simulink model "WaypointFollowing_Sim"  (R2021a)
settings: Solver=ode4  StartTime=0.0  StopTime=200  FixedStep=0.001  RelTol=1e-3
InitFcn:
  | Init_control;
values from neighbouring files (symbols this model uses):
  DEG2RAD = 0.0174533    [Init_control.m]
  Kd_PITCH_AngleRate = 0.001    [Init_control.m]
  Kd_ROLL_AngleRate = 0.001    [Init_control.m]
  Kd_YAW_AngleRate = 0.00    (= 0)    [Init_control.m]
  Ki_PITCH_AngleRate = 0.02    [Init_control.m]
  Ki_ROLL_AngleRate = 0.02    [Init_control.m]
  Ki_YAW_AngleRate = 0.01    [Init_control.m]
  Kp_PITCH_ANGLE = 6.5    [Init_control.m]
  Kp_PITCH_AngleRate = 0.1    [Init_control.m]
  Kp_ROLL_ANGLE = 6.5    [Init_control.m]
  Kp_ROLL_AngleRate = 0.1    [Init_control.m]
  Kp_YAW_AngleRate = 0.5    [Init_control.m]
  Kpxp = 1.0    (= 1)    [Init_control.m]
  Kpyp = 1.0    (= 1)    [Init_control.m]
  Kpzp = 4.0    (= 4)    [Init_control.m]
  Kvxd = 0.01    [Init_control.m]
  Kvxi = 0.4    [Init_control.m]
  Kvxp = 2.5    [Init_control.m]
  Kvyd = 0.01    [Init_control.m]
  Kvyi = 0.4    [Init_control.m]
  Kvyp = 2.5    [Init_control.m]
  Kvzd = 0.005    [Init_control.m]
  Kvzi = 0.01    [Init_control.m]
  Kvzp = 0.45    [Init_control.m]
  MAX_CONTROL_ANGLE_PITCH = 35    [Init_control.m]
  MAX_CONTROL_ANGLE_RATE_PITCH = 220    [Init_control.m]
  MAX_CONTROL_ANGLE_RATE_ROLL = 220    [Init_control.m]
  MAX_CONTROL_ANGLE_RATE_Y = 200    [Init_control.m]
  MAX_CONTROL_ANGLE_ROLL = 35    [Init_control.m]
  MAX_CONTROL_VELOCITY_XY = 5    [Init_control.m]
  MAX_CONTROL_VELOCITY_Z = 3    [Init_control.m]
  ModelInit_AngEuler = [0, 0, 0]    [Init_control.m]
  ModelInit_PosE = [0, 0, -100]    [Init_control.m]
  ModelInit_Rads = 0    [Init_control.m]
  ModelInit_RateB = [0, 0, 0]    [Init_control.m]
  ModelInit_VelB = [0, 0, 0]    [Init_control.m]
  Saturation_I_ah = 3.43    [Init_control.m]
  Saturation_I_az = 5    [Init_control.m]
  Saturation_I_RP_Max = 0.3    [Init_control.m]
  Saturation_I_RP_Min = -0.3    [Init_control.m]
  Saturation_I_Y_Max = 0.2    [Init_control.m]
  Saturation_I_Y_Min = -0.2    [Init_control.m]
  THR_HOVER = 0.609    [Init_control.m]
undefined symbols (not defined in the file or in its folder): DiscIntNeverNeededParam, earthRadius, ModelParam_envGravityAcc, ModelParam_motorCr, ModelParam_motorJm, ModelParam_motorT, ModelParam_motorWb, ModelParam_rotorCm, ModelParam_rotorCt, ModelParam_uavCCm, ModelParam_uavCd, ModelParam_uavJ, ModelParam_uavMass, ModelParam_uavR, Receive, Send
libraries: simulink x8, aerolibfltsims x3, sharedutil x2, aerolibanimutils x1
(part 2 of 2)

== matlab function WaypointFollowing_Sim/Quadcopter Dynamics/Rigid Model/Rigid-Body Kinematic Model /Quaternion to rotation matrix ==
  data: q input; Reb output
function Reb = fcn(q)
%Function description;
%  The rotation matrix of the Aircraft-Body Coordinate Frame (ABCF) to the
%  Earth-Fixed Coordinate Frame (EFCF) is obtained from the quaternions
Reb = [q(1)*q(1) + q(2)*q(2) - q(3)*q(3) - q(4)*q(4), 2*(q(2)*q(3) - q(1)*q(4)), 2*(q(2)*q(4) + q(1)*q(3))
           2*(q(2)*q(3) + q(1)*q(4)), q(1)*q(1) - q(2)*q(2) + q(3)*q(3) - q(4)*q(4), 2*(q(3)*q(4) - q(1)*q(2))
           2*(q(2)*q(4) - q(1)*q(3)), 2*(q(3)*q(4) + q(1)*q(2)), q(1)*q(1) - q(2)*q(2) - q(3)*q(3) + q(4)*q(4)];

== matlab function WaypointFollowing_Sim/Quadcopter Dynamics/Rigid Model/Rigid-Body Kinematic Model /Quaternions model ==
  data: pqr input; qdot output; q input
function qdot = fcn(pqr, q)
%Function description:
%  Quaternions model
qdot = 0.5*[0, -pqr(1), -pqr(2), -pqr(3); pqr(1), 0, pqr(3), -pqr(2); pqr(2), -pqr(3), 0, pqr(1); pqr(3), pqr(2), -pqr(1), 0]*q;

== matlab function WaypointFollowing_Sim/Control System/InputConditioning1/f1 ==
  data: in input; y output; hover input
function y = thr_curve(in, hover)
%Function description:
%  throttle curve. When the throttle is in the middle position, the output
%  is hovering throttle value.
%Input:
%  in: normalized throttle, range from 0 to 1
%  hover: hovering throttle value
%Output:
%  y: processed throttle value
if in < 0.5
	y=2 * in * hover;
else
	y=hover + 2 * (in - 0.5) * (1.0 - hover);
end

== matlab function WaypointFollowing_Sim/Control System/MATLAB Function1 ==
  data: reset_i output; ch3 input
function reset_i= fcn(ch3)
%Function description:
%  Reset Integral when throttle < 1250
if ch3<1250
    reset_i=[1 1 1 1];
else
    reset_i=[0 0 0 0];
end

== matlab function WaypointFollowing_Sim/Control System/InputConditioning/deadzone2 ==
  data: u input; y output
function y = fcn(u)
%Function description:
%  Control the range of the remote control input from RCMin to RCMax, and
%  set a dead zone with a dead zone size of ±deadZone. The output y is
%  normalized to 0~1.You can get the RC calibration parameters in QGC.
RCMin = 1100;
RCMax = 1900;
RCMid = (RCMin + RCMax)/2;
deadZoneRate = 0.05;
deadZone = deadZoneRate*(RCMax - RCMin);
k = 1/(RCMax - RCMid - deadZone);
% saturation
if(u < RCMin)
    u = RCMin;
elseif(u > RCMax)
    u = RCMax;
end
% dead zone and normalize
 if(u > RCMid + deadZone)
    y = (u-RCMid - deadZone)*k;
 elseif(u < RCMid - deadZone)
     y = (u - RCMid + deadZone)*k;
 else
     y = 0;
 end

 end

== matlab function WaypointFollowing_Sim/Control System/InputConditioning/deadzone1 ==
  data: u input; y output
function y = fcn(u)
%Function description:
%  Control the range of the remote control input from RCMin to RCMax, and
%  set a dead zone with a dead zone size of ±deadZone. The output y is
%  normalized to 0~1.You can get the RC calibration parameters in QGC.
RCMin = 1100;
RCMax = 1900;
RCMid = (RCMin + RCMax)/2;
deadZoneRate = 0.05;
deadZone = deadZoneRate*(RCMax - RCMin);
k = 1/(RCMax - RCMid - deadZone);
% saturation
if(u < RCMin)
    u = RCMin;
elseif(u > RCMax)
    u = RCMax;
end
% dead zone and normalize
 if(u > RCMid + deadZone)
    y = (u-RCMid - deadZone)*k;
 elseif(u < RCMid - deadZone)
     y = (u - RCMid + deadZone)*k;
 else
     y = 0;
 end

 end

== matlab function WaypointFollowing_Sim/Control System/InputConditioning1/deadzone1 ==
  data: u input; y output
function y = fcn(u)
%Function description:
%  Control the range of the remote control input from RCMin to RCMax, and
%  set a dead zone with a dead zone size of ±deadZone. The output y is
%  normalized to 0~1.You can get the RC calibration parameters in QGC.
RCMin = 1100;
RCMax = 1900;
RCMid = (RCMin + RCMax)/2;
deadZoneRate = 0.05;
deadZone = deadZoneRate*(RCMax - RCMin);
k = 1/(RCMax - RCMid - deadZone);
% saturation
if(u < RCMin)
    u = RCMin;
elseif(u > RCMax)
    u = RCMax;
end
% dead zone and normalize
 if(u > RCMid + deadZone)
    y = (u-RCMid - deadZone)*k;
 elseif(u < RCMid - deadZone)
     y = (u - RCMid + deadZone)*k;
 else
     y = 0;
 end

 end

== matlab function WaypointFollowing_Sim/Control System/InputConditioning1/deadzone2 ==
  data: u input; y output
function y = fcn(u)
%Function description:
%  Control the range of the remote control input from RCMin to RCMax, and
%  set a dead zone with a dead zone size of ±deadZone. The output y is
%  normalized to 0~1.You can get the RC calibration parameters in QGC.
RCMin = 1100;
RCMax = 1900;
RCMid = (RCMin + RCMax)/2;
deadZoneRate = 0.05;
deadZone = deadZoneRate*(RCMax - RCMin);
k = 1/(RCMax - RCMid - deadZone);
% saturation
if(u < RCMin)
    u = RCMin;
elseif(u > RCMax)
    u = RCMax;
end
% dead zone and normalize
 if(u > RCMid + deadZone)
    y = (u-RCMid - deadZone)*k;
 elseif(u < RCMid - deadZone)
     y = (u - RCMid + deadZone)*k;
 else
     y = 0;
 end

 end

== matlab function WaypointFollowing_Sim/Control System/InputConditioning1/deadzone3 ==
  data: u input; y output
function y = fcn(u)
%Function description:
%  Control the range of the remote control input from RCMin to RCMax, and
%  set a dead zone with a dead zone size of ±deadZone. The output y is
%  normalized to 0~1.You can get the RC calibration parameters in QGC.
RCMin = 1100;
RCMax = 1900;
RCMid = (RCMin + RCMax)/2;
deadZoneRate = 0.05;
deadZone = deadZoneRate*(RCMax - RCMin);
k = 1/(RCMax - RCMid - deadZone);
% saturation
if(u < RCMin)
    u = RCMin;
elseif(u > RCMax)
    u = RCMax;
end
% dead zone and normalize
 if(u > RCMid + deadZone)
    y = (u-RCMid - deadZone)*k;
 elseif(u < RCMid - deadZone)
     y = (u - RCMid + deadZone)*k;
 else
     y = 0;
 end

 end

== matlab function WaypointFollowing_Sim/Control System/InputConditioning/deadzone3 ==
  data: u input; y output
function y = fcn(u)
%Function description:
%  Control the range of the remote control input from RCMin to RCMax, and
%  set a dead zone with a dead zone size of ±deadZone. The output y is
%  normalized to 0~1.You can get the RC calibration parameters in QGC.
RCMin = 1100;
RCMax = 1900;
RCMid = (RCMin + RCMax)/2;
deadZoneRate = 0.05;
deadZone = deadZoneRate*(RCMax - RCMin);
k = 1/(RCMax - RCMid - deadZone);
% saturation
if(u < RCMin)
    u = RCMin;
elseif(u > RCMax)
    u = RCMax;
end
% dead zone and normalize
 if(u > RCMid + deadZone)
    y = (u-RCMid - deadZone)*k;
 elseif(u < RCMid - deadZone)
     y = (u - RCMid + deadZone)*k;
 else
     y = 0;
 end

 end

== matlab function WaypointFollowing_Sim/Control System/MATLAB Function2 ==
  settings: updateMethod=DISCRETE
  data: vxd input; vyd input; vx_d output; vy_d output; vz_d output; vzd input; x input; y input; z input; vx input; vy input; vz input; x_d output; y_d output; z_d output; waypoints input
function [vx_d, vy_d, vz_d, x_d, y_d, z_d]  = fcn(vxd, vyd, vzd, x, y, z, vx, vy, vz, waypoints)
%Function description:
%  position control implementation. When the desired velocity (specified by the remote controller) is < 0.001, 
%  and the current velocity is <6 m/s, the position hold is activated, and the desired position is the position at which 
%  the above condition is satisfied, the position loop and the velocity loop act simultaneously; when the condition 
%  is not satisfied, Only the velocity loop works.
%Input:
%  vxd, vyd, vzd: The desired velocity specified by the remote control
%  x, y, z: current position
%  vx, vy,vz: current velocity
%Output:
%  vx_d, vy_d, vz_d, x_d, y_d, z_d: desired velocity and position
persistent x1;
if isempty(x1)
    x1 = 0;
end
persistent y1;
if isempty(y1)
    y1 = 0;
end
persistent z1;
if isempty(z1)
    z1 = z;
end
persistent hold_x_flag;
if isempty(hold_x_flag)
    hold_x_flag = 0;
end
persistent hold_y_flag;
if isempty(hold_y_flag)
    hold_y_flag = 0;
end
persistent hold_z_flag;
if isempty(hold_z_flag)
    hold_z_flag = 0;
end

%% Guo 2021/4/11
persistent waypoint_1_flag;
if isempty(waypoint_1_flag)
    waypoint_1_flag = 0;
end

persistent waypoint_2_flag;
if isempty(waypoint_2_flag)
    waypoint_2_flag = 0;
end

persistent waypoint_3_flag;
if isempty(waypoint_3_flag)
    waypoint_3_flag = 0;
end

persistent waypoint_4_flag;
if isempty(waypoint_4_flag)
    waypoint_4_flag = 0;
end
if waypoint_1_flag == 0
    x1 = waypoints(1,1);
    y1 = waypoints(1,2);
    if abs(x-x1)<e && abs(y-y1)<e
        waypoint_1_flag = 1;
    end
elseif waypoint_2_flag == 0
    x1 = waypoints(2,1);
    y1 = waypoints(2,2);
    if abs(x-x1)<e && abs(y-y1)<e
        waypoint_2_flag = 1;
    end
elseif waypoint_3_flag == 0
    x1 = waypoints(3,1);
    y1 = waypoints(3,2);
    if abs(x-x1)<e && abs(y-y1)<e
        waypoint_3_flag = 1;
    end
elseif waypoint_4_flag == 0
    x1 = waypoints(4,1);
    y1 = waypoints(4,2);
    if abs(x-x1)<e && abs(y-y1)<e
        waypoint_4_flag = 1;
    end
else
    x1 = waypoints(1,1);
    y1 = waypoints(1,2);
    if abs(x-x1)<e && abs(y-y1)<e
        waypoint_1_flag = 0;
        waypoint_2_flag = 0;
        waypoint_3_flag = 0;
        waypoint_4_flag = 0;
    end
end
%%

if abs(vxd) < 0.001 && abs(vx) < 8
    hold_x = 1;
else
    hold_x = 0;
    hold_x_flag = 0;
end
if abs(vyd) < 0.001 && abs(vy) < 8
    hold_y = 1;
else
    hold_y = 0;
    hold_y_flag = 0;
end
if abs(vzd) < 0.001 && abs(vz) < 6
    hold_z = 1;
else
    hold_z = 0;
    hold_z_flag = 0;
end

if (hold_x > 0.5) && (hold_x_flag < 0.5)
    x1 = x;
    hold_x_flag = 1;
end
if (hold_y > 0.5) && (hold_y_flag < 0.5)
    y1 = y;
    hold_y_flag = 1;
end

% throttle in the middle position, hold the height
if (hold_z > 0.5) && (hold_z_flag < 0.5)
    z1 = z;
    hold_z_flag = 1;
end
%When the RC sticks(CH1, CH2, CH3, CH4) deviate from the middle dead zone range, the position is the current position. 
%The position controller only works with the velocity loop
if hold_x < 0.5
    x1 = x;
    hold_x_flag = 0;
end
if hold_y < 0.5
    y1 = y;
    hold_y_flag = 0;
end
if hold_z < 0.5
    z1 = z;
    hold_z_flag = 0;
end

e = 1;
%% Guo 2021/4/11
if waypoint_1_flag == 0
    x1 = waypoints(1,1);
    y1 = waypoints(1,2);
    if abs(x-x1)<e && abs(y-y1)<e
        waypoint_1_flag = 1;
    end
elseif waypoint_2_flag == 0
    x1 = waypoints(2,1);
    y1 = waypoints(2,2);
    if abs(x-x1)<e && abs(y-y1)<e
        waypoint_2_flag = 1;
    end
elseif waypoint_3_flag == 0
    x1 = waypoints(3,1);
    y1 = waypoints(3,2);
    if abs(x-x1)<e && abs(y-y1)<e
        waypoint_3_flag = 1;
    end
elseif waypoint_4_flag == 0
    x1 = waypoints(4,1);
    y1 = waypoints(4,2);
    if abs(x-x1)<e && abs(y-y1)<e
        waypoint_4_flag = 1;
    end
else
    x1 = waypoints(1,1);
    y1 = waypoints(1,2);
    if abs(x-x1)<e && abs(y-y1)<e
        waypoint_1_flag = 0;
        waypoint_2_flag = 0;
        waypoint_3_flag = 0;
        waypoint_4_flag = 0;
    end
end
%%
vx_d = vxd; vy_d = vyd; vz_d = vzd;

x_d = x1;
y_d = y1;
z_d = z1;
